simulink model "TST_CrCtl_StM"  (R2016b)
settings: Solver=FixedStepDiscrete  StartTime=0.0  StopTime=simTime  FixedStep=sampleTime  RelTol=1e-3
values from neighbouring files (symbols this model uses):
  testCase = 1    [initTST_CrCtl_StM_001.m]    (also in initTST_CrCtl_StM_002.m = 2)
libraries: simulink x31, UnitTest_Lib x18
(part 2 of 2)

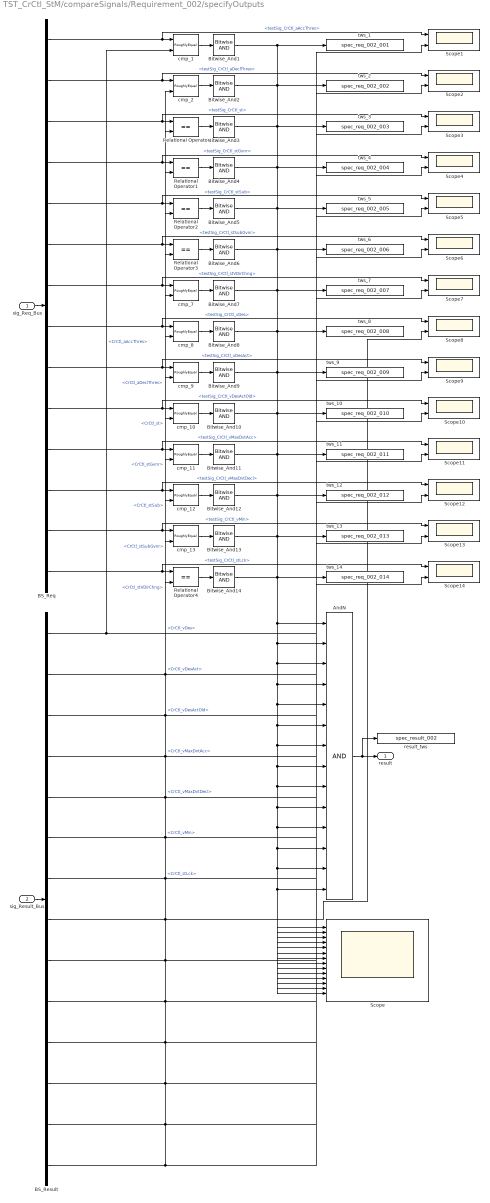
== system TST_CrCtl_StM/compareSignals/Requirement_002/specifyOutputs ==
  sig_Req_Bus : Inport
  sig_Result_Bus : Inport  Port=2
  AndN : Logic  Inputs=14
  BS_Req : BusSelector  OutputSignals=testSig_CrCtl_aAccThres,testSig_CrCtl_aDeclThres,testSig_CrCtl_st,testSig_CrCtl_stGvnr,testSig_CrCtl_stSub,testSig_CrCtl_stSubGvnr,testSig_CrCtl_stVDirChng,testSig_CrCtl_vDes,testSig_CrCtl_vDesAct,testSig_CrCtl_vDesActOld,testSig_CrCtl_vMaxDvtAcc,testSig_CrCtl_vMaxDvtDecl,testSig_CrCtl_vMin,testSig_CrCtl_stLck
  BS_Result : BusSelector  OutputSignals=CrCtl_aAccThres,CrCtl_aDeclThres,CrCtl_st,CrCtl_stGvnr,CrCtl_stSub,CrCtl_stSubGvnr,CrCtl_stVDirChng,CrCtl_vDes,CrCtl_vDesAct,CrCtl_vDesActOld,CrCtl_vMaxDvtAcc,CrCtl_vMaxDvtDecl,CrCtl_vMin,CrCtl_stLck
  Bitwise_And{1..14} (14 alike) : simulink/Logic and Bit Operations/Bitwise Operator  logicop=AND  UseBitMask=off  BitMask=bin2dec('11011001')  BitMaskRealWorld=Stored Integer
  Relational Operator{,1..4} (5 alike) : RelationalOperator  Operator===  OutDataTypeStr=boolean  RndMeth=Simplest
  Scope : Scope  NumInputPorts=14
  Scope{1..14} (14 alike) : Scope  NumInputPorts=2
  cmp_{1..2,7..13} (9 alike) : UnitTest_Lib/RoughlyEqual  slope=0.1
  result_tws : ToWorkspace  VariableName=spec_result_002
  tws_1 : ToWorkspace  VariableName=spec_req_002_001
  tws_10 : ToWorkspace  VariableName=spec_req_002_010
  tws_11 : ToWorkspace  VariableName=spec_req_002_011
  tws_12 : ToWorkspace  VariableName=spec_req_002_012
  tws_13 : ToWorkspace  VariableName=spec_req_002_013
  tws_14 : ToWorkspace  VariableName=spec_req_002_014
  tws_2 : ToWorkspace  VariableName=spec_req_002_002
  tws_3 : ToWorkspace  VariableName=spec_req_002_003
  tws_4 : ToWorkspace  VariableName=spec_req_002_004
  tws_5 : ToWorkspace  VariableName=spec_req_002_005
  tws_6 : ToWorkspace  VariableName=spec_req_002_006
  tws_7 : ToWorkspace  VariableName=spec_req_002_007
  tws_8 : ToWorkspace  VariableName=spec_req_002_008
  tws_9 : ToWorkspace  VariableName=spec_req_002_009
  result : Outport
  wires:
  sig_Req_Bus/1 -> BS_Req/1
  sig_Result_Bus/1 -> BS_Result/1
  AndN/1 -> result/1, result_tws/1
  BS_Req/1 -> cmp_1/1, Scope1/1  "<testSig_CrCtl_aAccThres>"
  BS_Result/1 -> cmp_1/2, Scope1/2  "<CrCtl_aAccThres>"
  cmp_1/1 -> Bitwise_And1/1
  Bitwise_And1/1 -> AndN/1, Scope/1, tws_1/1
  BS_Req/2 -> cmp_2/1, Scope2/1  "<testSig_CrCtl_aDeclThres>"
  BS_Result/2 -> cmp_2/2, Scope2/2  "<CrCtl_aDeclThres>"
  cmp_2/1 -> Bitwise_And2/1
  Bitwise_And2/1 -> AndN/2, Scope/2, tws_2/1
  BS_Req/3 -> Relational Operator/1, Scope3/1  "<testSig_CrCtl_st>"
  BS_Result/3 -> Relational Operator/2, Scope3/2  "<CrCtl_st>"
  Relational Operator/1 -> Bitwise_And3/1
  Bitwise_And3/1 -> AndN/3, Scope/3, tws_3/1
  BS_Req/4 -> Relational Operator1/1, Scope4/1  "<testSig_CrCtl_stGvnr>"
  BS_Result/4 -> Relational Operator1/2, Scope4/2  "<CrCtl_stGvnr>"
  Relational Operator1/1 -> Bitwise_And4/1
  Bitwise_And4/1 -> AndN/4, Scope/4, tws_4/1
  BS_Req/5 -> Relational Operator2/1, Scope5/1  "<testSig_CrCtl_stSub>"
  BS_Result/5 -> Relational Operator2/2, Scope5/2  "<CrCtl_stSub>"
  Relational Operator2/1 -> Bitwise_And5/1
  Bitwise_And5/1 -> AndN/5, Scope/5, tws_5/1
  BS_Req/6 -> Relational Operator3/1, Scope6/1  "<testSig_CrCtl_stSubGvnr>"
  BS_Result/6 -> Relational Operator3/2, Scope6/2  "<CrCtl_stSubGvnr>"
  Relational Operator3/1 -> Bitwise_And6/1
  Bitwise_And6/1 -> AndN/6, Scope/6, tws_6/1
  BS_Req/7 -> cmp_7/1, Scope7/1  "<testSig_CrCtl_stVDirChng>"
  BS_Result/7 -> cmp_7/2, Scope7/2  "<CrCtl_stVDirChng>"
  cmp_7/1 -> Bitwise_And7/1
  Bitwise_And7/1 -> AndN/7, Scope/7, tws_7/1
  BS_Req/8 -> cmp_8/1, Scope8/1  "<testSig_CrCtl_vDes>"
  BS_Result/8 -> cmp_8/2, Scope8/2  "<CrCtl_vDes>"
  cmp_8/1 -> Bitwise_And8/1
  Bitwise_And8/1 -> AndN/8, Scope/8, tws_8/1
  BS_Req/9 -> cmp_9/1, Scope9/1  "<testSig_CrCtl_vDesAct>"
  BS_Result/9 -> cmp_9/2, Scope9/2  "<CrCtl_vDesAct>"
  cmp_9/1 -> Bitwise_And9/1
  Bitwise_And9/1 -> AndN/9, Scope/9, tws_9/1
  BS_Req/10 -> cmp_10/1, Scope10/1  "<testSig_CrCtl_vDesActOld>"
  BS_Result/10 -> cmp_10/2, Scope10/2  "<CrCtl_vDesActOld>"
  cmp_10/1 -> Bitwise_And10/1
  Bitwise_And10/1 -> AndN/10, Scope/10, tws_10/1
  BS_Req/11 -> cmp_11/1, Scope11/1  "<testSig_CrCtl_vMaxDvtAcc>"
  BS_Result/11 -> cmp_11/2, Scope11/2  "<CrCtl_vMaxDvtAcc>"
  cmp_11/1 -> Bitwise_And11/1
  Bitwise_And11/1 -> AndN/11, Scope/11, tws_11/1
  BS_Req/12 -> cmp_12/1, Scope12/1  "<testSig_CrCtl_vMaxDvtDecl>"
  BS_Result/12 -> cmp_12/2, Scope12/2  "<CrCtl_vMaxDvtDecl>"
  cmp_12/1 -> Bitwise_And12/1
  Bitwise_And12/1 -> AndN/12, Scope/12, tws_12/1
  BS_Req/13 -> cmp_13/1, Scope13/1  "<testSig_CrCtl_vMin>"
  BS_Result/13 -> cmp_13/2, Scope13/2  "<CrCtl_vMin>"
  cmp_13/1 -> Bitwise_And13/1
  Bitwise_And13/1 -> AndN/13, Scope/13, tws_13/1
  BS_Req/14 -> Relational Operator4/1, Scope14/1  "<testSig_CrCtl_stLck>"
  BS_Result/14 -> Relational Operator4/2, Scope14/2  "<CrCtl_stLck>"
  Relational Operator4/1 -> Bitwise_And14/1
  Bitwise_And14/1 -> AndN/14, Scope/14, tws_14/1
